simulink model "DOB_demo"  (R2024a)
settings: Solver=VariableStepAuto  StartTime=0.0  StopTime=15.0  RelTol=1e-3
settings Model: Creator=XieXW  LastModifiedBy=XieXW

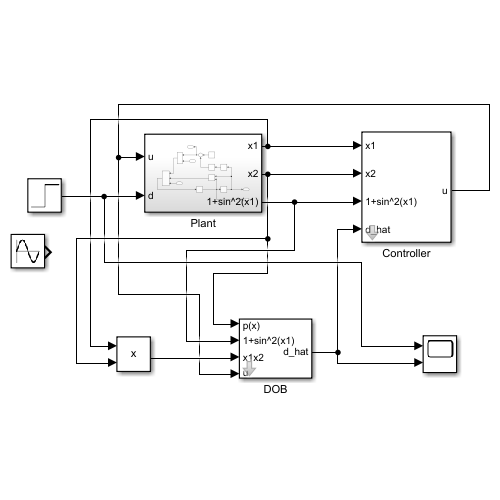
[thumbnail: Simulink's stored preview of the top-level diagram]
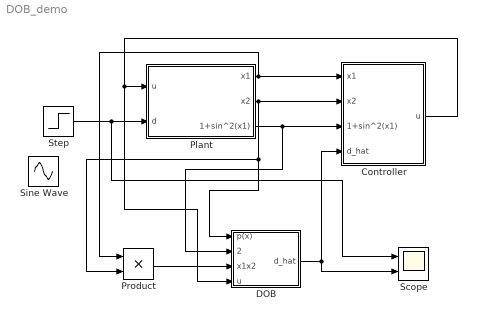
== system DOB_demo ==
  Controller : Subsystem  mask{k1=1, k2=1}
      mask DialogControl ParameterGroupVar Prompt: 参数
  DOB : Subsystem  mask{c=10}
      mask prompts: c "观测器增益l(x)"
      mask DialogControl ParameterGroupVar Prompt: 参数
  Plant : Subsystem
  Product : Product
  Scope : Scope  NumInputPorts=2
  Sine Wave : Sin  SampleTime=0
  Step : Step  Time=6  Before=2  After=6  SampleTime=0
  wires:
  Plant/1(x1) -> Product/1, Controller/1(x1)
  Plant/2(x2) -> Product/2, DOB/1(p(x)), Controller/2(x2)
  Plant/3(1+sin^2(x1)) -> DOB/2(1+sin^2(x1)), Controller/3(1+sin^2(x1))
  Controller/1(u) -> Plant/1(u), DOB/4(u)
  DOB/1(d_hat) -> Scope/2, Controller/4(d_hat)
  Product/1 -> DOB/3(x1x2)
  Step/1 -> Scope/1, Plant/2(d)

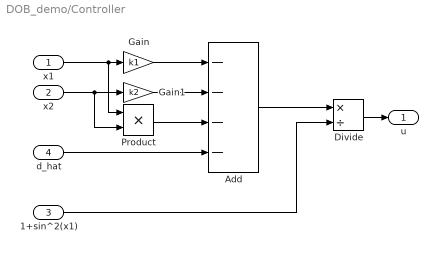
== system DOB_demo/Controller ==
  x1 : Inport
  x2 : Inport  Port=2
  1+sin^2(x1) : Inport  Port=3
  d_hat : Inport  Port=4
  Add : Sum  Inputs=----
  Divide : Product  Inputs=*/
  Gain : Gain  Gain=k1
  Gain1 : Gain  Gain=k2
  Product : Product
  u : Outport
  wires:
  x1/1 -> Product/1, Gain/1
  x2/1 -> Product/2, Gain1/1
  Gain/1 -> Add/1
  Gain1/1 -> Add/2
  Product/1 -> Add/3
  d_hat/1 -> Add/4
  Add/1 -> Divide/1
  1+sin^2(x1)/1 -> Divide/2
  Divide/1 -> u/1

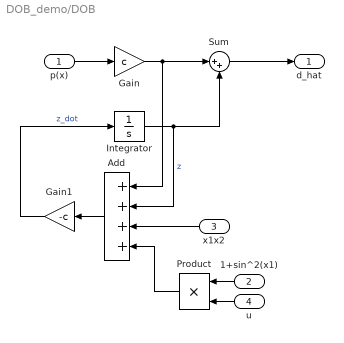
== system DOB_demo/DOB ==
  p(x) : Inport
  1+sin^2(x1) : Inport  Port=2
  x1x2 : Inport  Port=3
  u : Inport  Port=4
  Add : Sum  Inputs=++++
  Gain : Gain  Gain=c
  Gain1 : Gain  Gain=-c
  Integrator : Integrator
  Product : Product
  Sum : Sum  Inputs=|++
  d_hat : Outport
  wires:
  p(x)/1 -> Gain/1
  Gain/1 -> Add/1, Sum/1
  Sum/1 -> d_hat/1
  Integrator/1 -> Add/2, Sum/2  "z"
  Gain1/1 -> Integrator/1  "z_dot"
  x1x2/1 -> Add/3
  u/1 -> Product/2
  1+sin^2(x1)/1 -> Product/1
  Product/1 -> Add/4
  Add/1 -> Gain1/1

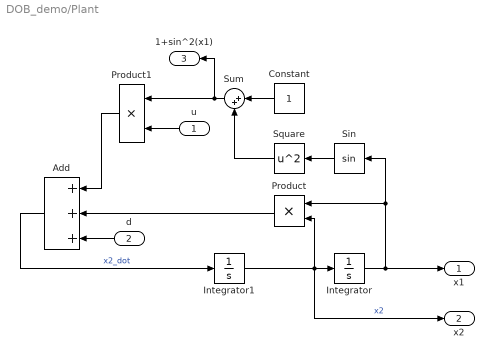
== system DOB_demo/Plant ==
  u : Inport
  d : Inport  Port=2
  Add : Sum  Inputs=+++
  Constant : Constant
  Integrator : Integrator
  Integrator1 : Integrator
  Product : Product
  Product1 : Product
  Sin : Trigonometry
  Square : Math  Operator=square
  Sum : Sum  Inputs=|++
  x1 : Outport
  x2 : Outport  Port=2
  1+sin^2(x1) : Outport  Port=3
  wires:
  Integrator/1 -> Sin/1, Product/1, x1/1
  Integrator1/1 -> x2/1, Product/2, Integrator/1  "x2"
  Add/1 -> Integrator1/1  "x2_dot"
  Constant/1 -> Sum/1
  Sin/1 -> Square/1
  Square/1 -> Sum/2
  Sum/1 -> 1+sin^2(x1)/1, Product1/1
  u/1 -> Product1/2
  Product1/1 -> Add/1
  Product/1 -> Add/2
  d/1 -> Add/3
